simulink model "sunSeek_test"  (R2018b)
settings: Solver=VariableStepAuto  StartTime=0.0  StopTime=600  RelTol=1e-3
libraries: pd_processing_lib x1, quat_kinematics_lib x1, rigid_body_dynamics_lib x1, solar_panels_lib x1, sunSeek_lib x1, sun_sensor_lib x1, MEKF_Conversion_lib x1
settings Model: Creator=Taylor  LastModifiedBy=Taylor

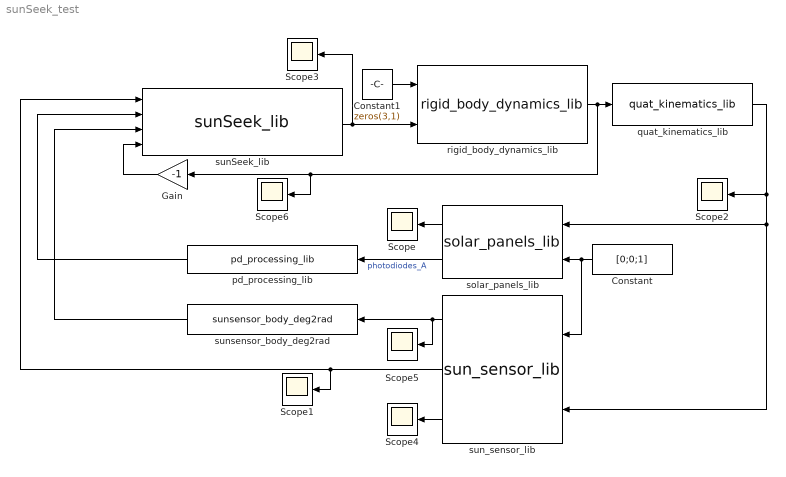
== system sunSeek_test ==
  Constant : Constant  Value=[0;0;1]
  Constant1 : Constant  Value=zeros(3,1)
  Gain : Gain  Gain=-1
  Scope{,1..6} (7 alike) : Scope
  pd_processing_lib : pd_processing_lib/pd_processing_lib  SystemSampleTime=-1
  quat_kinematics_lib : quat_kinematics_lib/quat_kinematics_lib  SystemSampleTime=-1
  rigid_body_dynamics_lib : rigid_body_dynamics_lib/rigid_body_dynamics_lib  SystemSampleTime=-1
  solar_panels_lib : solar_panels_lib/solar_panels_lib  SystemSampleTime=-1
  sunSeek_lib : sunSeek_lib/sunSeek_lib  SystemSampleTime=-1
  "sun_sensor_lib " : sun_sensor_lib/sun_sensor_lib   SystemSampleTime=-1
  sunsensor_body_deg2rad : MEKF_Conversion_lib/Conversion_lib/sunsensor_body_deg2rad  SystemSampleTime=-1
  wires:
  rigid_body_dynamics_lib/1 -> Scope6/1, Gain/1, quat_kinematics_lib/1
  Constant1/1 -> rigid_body_dynamics_lib/1
  solar_panels_lib/2 -> pd_processing_lib/1  "photodiodes_A"
  solar_panels_lib/1 -> Scope/1
  Constant/1 -> "sun_sensor_lib "/1, solar_panels_lib/2
  quat_kinematics_lib/1 -> "sun_sensor_lib "/2, solar_panels_lib/1, Scope2/1
  "sun_sensor_lib "/3 -> Scope4/1
  "sun_sensor_lib "/2 -> Scope1/1, sunSeek_lib/1
  "sun_sensor_lib "/1 -> sunsensor_body_deg2rad/1, Scope5/1
  sunSeek_lib/1 -> rigid_body_dynamics_lib/2, Scope3/1
  pd_processing_lib/1 -> sunSeek_lib/2
  sunsensor_body_deg2rad/1 -> sunSeek_lib/3
  Gain/1 -> sunSeek_lib/4
